simulink model "stm32f0_clcd_demo"  (Simulink 7.3)
settings: Solver=ode3  SolverMode=SingleTasking  StartTime=0.0  StopTime=10.0  RelTol=1e-3
PreLoadFcn:
  | waijung.modelPreload; % Required for working with Waijung Blockset. Do not remove.
undefined symbols (not defined in the file): LQFP48, STM32F072CB
libraries: simulink x34, waijung_soft_i2c_lib x12, waijung_string_manipulate x4, stm32f0_device_config_lib x1
CloseFcn:
  | waijung.modelClose; % Required for working with Waijung Blockset. Do not remove.
settings Model: Creator=Krisada  LastModifiedBy=Krisada
settings OptimizationCC: OptimizeModelRefInitCode=on  LifeSpan=1
settings HardwareCC: ProdEndianess=LittleEndian  ProdHWDeviceType=ARM Compatible->Cortex - M0  TargetEndianess=LittleEndian  TargetHWDeviceType=ARM Compatible->Cortex - M0
settings RTWCC: SystemTargetFile=stm32f0.tlc  GenerateMakefile=off  TemplateMakefile=ert_default_tmf  Description=STM32F0 Target  ProcessScript=stm32f0_make_rtw_hook
settings CodeAppCC: IgnoreCustomStorageClasses=off
settings STFCustomTargetCC: ModelReferenceCompliant=off  CombineOutputUpdateFcns=on  ERTCustomFileBanners=on  SupportContinuousTime=off  SupportNonInlinedSFcns=off  SystemTargetFile=stm32f0.tlc
settings ERTTargetCC: MultiwordLength=2048  ModelReferenceCompliant=off  ParMdlRefBuildCompliant=off  CompOptLevelCompliant=off  ERTFirstTimeCompliant=off  ModelStepFunctionPrototypeControlCompliant=off  CPPClassGenCompliant=off  InlinedParameterPlacement=NonHierarchical  ERTSrcFileBannerTemplate=stm32f0_code_template.cgt  ERTHdrFileBannerTemplate=stm32f0_code_template.cgt  ERTDataSrcFileTemplate=stm32f0_code_template.cgt  ERTDataHdrFileTemplate=stm32f0_code_template.cgt  ERTCustomFileTemplate=stm32f0_file_process.tlc

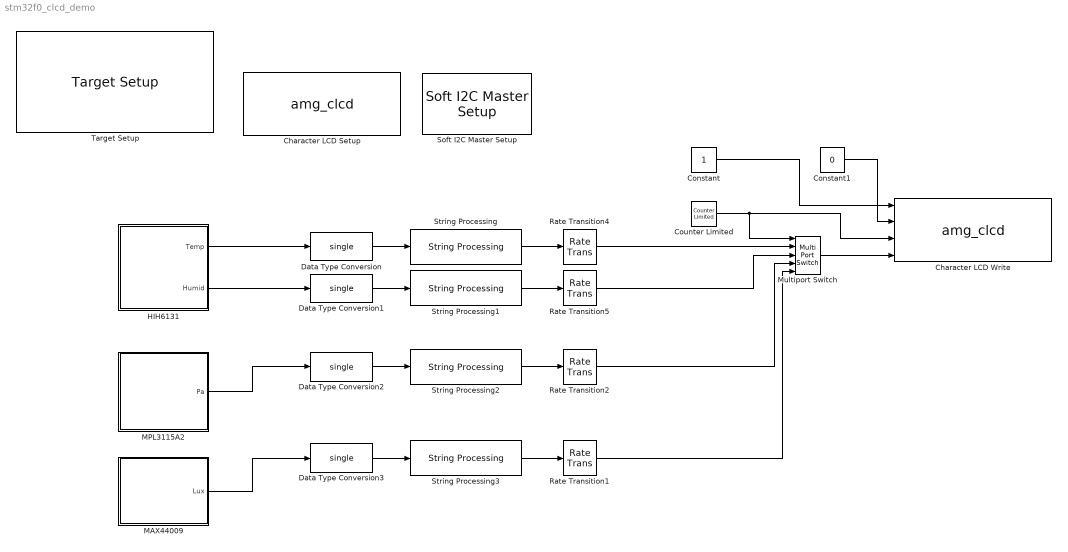
== system stm32f0_clcd_demo ==
  Character LCD Setup : S-Function  FunctionName=amg_clcd  Parameters=module,configuration,inputtypearray,outputtypearray,confstr,sampletime,sampletimestr,blockid  EnableBusSupport=off  mask(amg_clcd){configuration=Setup, module=1, model=amg CLCD Std, interface=4-bits, linecount=4, columncount=16, gpiotype=Push-pull, controlport=B, control_rs=2, control_rw=10, control_en=11, dataport=B, data0=12, data1=13, data2=0, data3=1, usestringbuffer=off, stringbuffer=<empty>, varname=, inputtypearray=[0], outputtypearray=[0], confstr=["4","4","16","PP","B","2","11","10","","B","","","","","12","13","0","1","0","","0","1","0","0","0","0","0","0","0","stm32f0"], sampletime=-1, sampletimestr=0.1, blockid=CharacterLCDSetup}
      mask prompts: model "LCD model:"; linecount "Number of lines (2 or 4):"; columncount "Number of columns (16 or 20):"; gpiotype "GPIO Output type:"; controlport "GPIO control port:"; control_rs "GPIO control pin, RS:"; control_rw "GPIO control pin, RW:"; control_en "GPIO control pin, EN:"; dataport "GPIO data D[7:4] port"; data0 "GPIO data pin, D4:"; data1 "GPIO data pin, D5:"; data2 "GPIO data pin, D6:"; data3 "GPIO data pin, D7:"; usestringbuffer "Use string buffer"; stringbuffer "String buffer"; varname "Variable name"; inputtypearray "Input type array"; outputtypearray "Output type array"; confstr "Configuration string"; sampletime "Sample time (sec)"; sampletimestr "Compiled sample time (sec) in string"
      mask init:
      | amg_clcd_callback('init');
      mask Help: web(fullfile(waijungdocroot,'amg_clcd_setup.htm'), '-browser')
      mask StyleString: popup(Setup|Transaction),popup(1|2|3|4),popup(amg CLCD Std),popup(4-bits),edit,edit,popup(Push-pull|Open-drain),popup(A|B|C|D|E|F|G|H|I),popup(0|1|2|3|4|5|6|7|8|9|10|11|12|13|14|15),popup(0|1|2|3|4|5|6|7|8|9|10|11|12|13|14|15),popup(0|1|2|3|4|5|6|7|8|9|10|11|12|13|14|15),popup(A|B|C|D|E|F|G|H|I),popup(0|1|2|3|4|5|6|7|8|9|10|11|12|13|14|15),popup(0|1|2|3|4|5|6|7|8|9|10|11|12|13|14|15),popup(0|1|2|3|4|5|6|7|8|9|10|11|12|13|14|15),popup(0|1|2|3|4|5|6|7|8|9|10|11|12|13|14|15),checkbox,popup(<empty>),edit,edit,edit,edit,edit,edit,edit
      mask CallbackString: amg_clcd_callback('configuration');||||||||||||||||amg_clcd_callback('usestringbuffer');||amg_clcd_callback('varname');|||amg_clcd_callback('confstr');|amg_clcd_callback('sampletime');|amg_clcd_callback('sampletimestr');|amg_clcd_callback('blockid');
      mask Display: text(0.5, 0.5, 'Module: CLCD1 (Setup)\nInterface: 4-bits\nCntrl: B2/B10/B11\nD[7:4]: B12/B13/B0/B1\nTs (sec): 0.1','ver','middle','hor','center');
  Character LCD Write : S-Function  FunctionName=amg_clcd  Parameters=module,configuration,inputtypearray,outputtypearray,confstr,sampletime,sampletimestr,blockid  EnableBusSupport=off  mask(amg_clcd){configuration=Transaction, module=1, model=amg CLCD Std, interface=4-bits, linecount=4, columncount=20, gpiotype=Push-pull, controlport=E, control_rs=15, control_rw=13, control_en=11, dataport=A, data0=7, data1=5, data2=3, data3=1, usestringbuffer=off, stringbuffer=<empty>, varname=, inputtypearray=[4 -1 -1 -1 -1], outputtypearray=[0], confstr=["4","4","20","PP","E","15","11","13","","A","","","","","7","5","3","1","0","","1","0","0","0","1","0","0","0","0","stm32f0"], sampletime=-1, sampletimestr=0.1, blockid=CharacterLCDWrite}
      mask prompts: model "LCD model:"; linecount "Number of lines:"; columncount "Number of columns:"; gpiotype "GPIO Output type:"; controlport "GPIO control port:"; control_rs "GPIO control pin, RS:"; control_rw "GPIO control pin, RW:"; control_en "GPIO control pin, EN:"; dataport "GPIO data D[7:4] port"; data0 "GPIO data pin, D4:"; data1 "GPIO data pin, D5:"; data2 "GPIO data pin, D6:"; data3 "GPIO data pin, D7:"; usestringbuffer "Use string buffer"; stringbuffer "String buffer"; varname "Variable name"; inputtypearray "Input type array"; outputtypearray "Output type array"; confstr "Configuration string"; sampletime "Sample time (sec)"; sampletimestr "Compiled sample time (sec) in string"
      mask help:
      | Note for cmd:
      | 1 - Clear specified LCD line display before write data to LCD.
      | Otherwise (e.g. 0) - Write data without clearing LCD Line.
      |
      | Position:
      | x = 0, First Character (from left to right)
      | y = 0, Top Line
      mask init:
      | amg_clcd_callback('init');
      mask Help: web(fullfile(waijungdocroot,'amg_clcd_write.htm'), '-browser')
      mask StyleString: popup(Setup|Transaction),popup(1|2|3|4),popup(amg CLCD Std),popup(4-bits),edit,edit,popup(Push-pull|Open-drain),popup(A|B|C|D|E|F|G|H|I),popup(0|1|2|3|4|5|6|7|8|9|10|11|12|13|14|15),popup(0|1|2|3|4|5|6|7|8|9|10|11|12|13|14|15),popup(0|1|2|3|4|5|6|7|8|9|10|11|12|13|14|15),popup(A|B|C|D|E|F|G|H|I),popup(0|1|2|3|4|5|6|7|8|9|10|11|12|13|14|15),popup(0|1|2|3|4|5|6|7|8|9|10|11|12|13|14|15),popup(0|1|2|3|4|5|6|7|8|9|10|11|12|13|14|15),popup(0|1|2|3|4|5|6|7|8|9|10|11|12|13|14|15),checkbox,popup(<empty>),edit,edit,edit,edit,edit,edit,edit
      mask CallbackString: amg_clcd_callback('configuration');||||||||||||||||amg_clcd_callback('usestringbuffer');||amg_clcd_callback('varname');|||amg_clcd_callback('confstr');|amg_clcd_callback('sampletime');|amg_clcd_callback('sampletimestr');|amg_clcd_callback('blockid');
      mask Display: text(0.5, 0.5, 'Module: CLCD1 (Write)\nTs (sec): 0.1','ver','middle','hor','center');port_label('input', 1,'cmd');port_label('input', 2,'xpos');port_label('input', 3,'ypos');port_label('input', 4,'str');
  Constant : Constant  OutDataType=fixdt(1, 16)  OutScaling=2^0
  Constant1 : Constant  Value=0  OutDataType=fixdt(1, 16)  OutScaling=2^0
  Counter Limited : simulink/Sources/Counter Limited  SystemSampleTime=-1  uplimit=3  tsamp=-1
  Data Type Conversion{,1..3} (4 alike) : DataTypeConversion  OutDataTypeMode=single  OutDataType=fixdt(1, 16)  OutScaling=2^0  OutDataTypeStr=single
  HIH6131 : Subsystem
  MAX44009 : Subsystem
  MPL3115A2 : Subsystem
  Multiport Switch : MultiPortSwitch  Inputs=4  zeroidx=on  OutDataType=fixdt(1, 16)  OutScaling=2^0
  Rate Transition{1..2,4..5} (4 alike) : RateTransition
  Soft I2C Master Setup : waijung_soft_i2c_lib/Soft I2C Master Setup  conf=Setup  targetname=stm32f0  module=1  transfer=Blocking  clk=250  timeout=25  sdapins='B7'  sclpins='B6'  writecount=1  readcount=1  waittime=0  forcestop=off  portpinstr=0  sampletime=-1  blockid=SoftI2CMasterSetup  inputporttype=[]  inputportwidth=[]  inputportlabel={}  outputporttype=[]  outputportwidth=[]  outputportlabel={}  compat=0  optionstring="[\"1\",\"250000\",\"3\",\"2\",\"1\",\"1\",\"25\",\"\",\"\",\"\",\"0\",\"1\",\"0\",\"0\",\"0\",\"0\",\"0\",\"0\",\"0\",\"\",\"1\",\"B\",\"7\",\"B\",\"6\"]"
  String Processing : waijung_string_manipulate/String Processing  conf=processing  stringfunction=sprintf  stringformat='Temp:%1.2f'  begindelimiter=''  enddelimiter=''  buffersize=16  enablestatus=off  portpinstr=0  sampletime=inf  blockid=StringProcessing  inputporttype=[-1]  inputportwidth=[1]  inputportlabel={'%f'}  outputporttype=[3]  outputportwidth=[16]  outputportlabel={'Output'}  compat=0  optionstring=[]  datatypestring="[\"float\"]"
  String Processing1 : waijung_string_manipulate/String Processing  conf=processing  stringfunction=sprintf  stringformat='Humid:%1.2f'  begindelimiter=''  enddelimiter=''  buffersize=16  enablestatus=off  portpinstr=0  sampletime=inf  blockid=StringProcessing1  inputporttype=[-1]  inputportwidth=[1]  inputportlabel={'%f'}  outputporttype=[3]  outputportwidth=[16]  outputportlabel={'Output'}  compat=0  optionstring=[]  datatypestring="[\"float\"]"
  String Processing2 : waijung_string_manipulate/String Processing  conf=processing  stringfunction=sprintf  stringformat='Pa: %1.2f'  begindelimiter=''  enddelimiter=''  buffersize=16  enablestatus=off  portpinstr=0  sampletime=inf  blockid=StringProcessing2  inputporttype=[-1]  inputportwidth=[1]  inputportlabel={'%f'}  outputporttype=[3]  outputportwidth=[16]  outputportlabel={'Output'}  compat=0  optionstring=[]  datatypestring="[\"float\"]"
  String Processing3 : waijung_string_manipulate/String Processing  conf=processing  stringfunction=sprintf  stringformat='Lux: %1.2f'  begindelimiter=''  enddelimiter=''  buffersize=16  enablestatus=off  portpinstr=0  sampletime=inf  blockid=StringProcessing3  inputporttype=[-1]  inputportwidth=[1]  inputportlabel={'%f'}  outputporttype=[3]  outputportwidth=[16]  outputportlabel={'Output'}  compat=0  optionstring=[]  datatypestring="[\"float\"]"
  Target Setup : stm32f0_device_config_lib/Target Setup  Priority=100  compiler=GNU ARM  previous_compiler=GNU ARM  mcu=STM32F072CB (LQFP48)  mcustr=STM32F072CB  stdlib=STM32F072  clockconfig=FiO MOTE-ST Default (HSEOSC-8MHz/HCLK-48MHz)  system_stm32f0xx_c_path=F:\trunk\targets\stm32f0_target\stm32f0\utils\STM32F0xx_AN4055\stm32f0_default\hse8mhz_pll_hclk48mhz  showmemoryconfiguration=on  stacksize=0x400  heapsize=0x200  enableautocompiledownload=on  fullchiperase=off  programmerinterface=aMG USB Connect  editctrlstr=on  compilercontrolstr=$(patsubst %, -I%, .) -mcpu=cortex-m0 -mthumb -mabi=aapcs -Wall -O3 -mfloat-abi=soft -ffunction-sections -fdata-sections -fno-strict-aliasing -fno-builtin --short-enums  assemblercontrolstr=$(patsubst %, -I%, .) -mcpu=cortex-m0 -mtune=cortex-m0 -mthumb -Wall -O3 -Wa,-amhls=$(<:.s=.lst) -D__STACK_SIZE=$(STACK_SIZE) -D__HEAP_SIZE=$(HEAP_SIZE)  linkercontrolstr="-T$(LD_SCRIPT) -Wl,-Map=$(MAP),--cref,--no-warn-mismatch -mcpu=cortex-m0 -mthumb  -Wall -O3 -mabi=aapcs -lc -specs=nosys.specs"  runafterdownload=on  execprofile=None  profileruart=3  profilerbaud=500000  profilertxpin=Not used  profilerinitstr=0.1,48000000,4800000,500000,0  manualsetsampletime=off  sampletime=0.1  blockid=TargetSetup  systickreloadvalue=4800000  hseval=8000000  lastprofileruart=3  hclk=48000000  flashorigin=0x8000000  flashlength=128k  ramorigin=0x20000000  ramlength=16k  useextram=off
  wires:
  Data Type Conversion/1 -> String Processing/1
  Data Type Conversion1/1 -> String Processing1/1
  Data Type Conversion3/1 -> String Processing3/1
  String Processing/1 -> Rate Transition4/1
  String Processing1/1 -> Rate Transition5/1
  String Processing3/1 -> Rate Transition1/1
  Counter Limited/1 -> Multiport Switch/1, Character LCD Write/3
  Multiport Switch/1 -> Character LCD Write/4
  Constant/1 -> Character LCD Write/1
  Constant1/1 -> Character LCD Write/2
  Rate Transition4/1 -> Multiport Switch/2
  Rate Transition5/1 -> Multiport Switch/3
  Data Type Conversion2/1 -> String Processing2/1
  String Processing2/1 -> Rate Transition2/1
  Rate Transition2/1 -> Multiport Switch/4
  Rate Transition1/1 -> Multiport Switch/5
  HIH6131/1(Temp) -> Data Type Conversion/1
  HIH6131/2(Humid) -> Data Type Conversion1/1
  MPL3115A2/1(Pa) -> Data Type Conversion2/1
  MAX44009/1(Lux) -> Data Type Conversion3/1

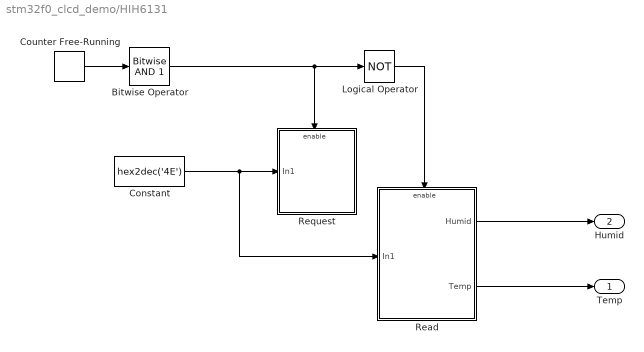
== system stm32f0_clcd_demo/HIH6131 ==
  Bitwise Operator : simulink/Logic and Bit Operations/Bitwise Operator  logicop=AND  UseBitMask=on  BitMask=1  BitMaskRealWorld=Stored Integer
  Constant : Constant  Value=hex2dec('4E')  OutDataTypeMode=uint8  OutDataType=fixdt(1, 16)  OutScaling=2^0  OutDataTypeStr=uint8  SampleTime=0.5
  Counter Free-Running : simulink/Sources/Counter Free-Running  SystemSampleTime=-1  NumBits=16  tsamp=-1
  Logical Operator : Logic  Operator=NOT  AllPortsSameDT=off  OutDataTypeMode=boolean  LogicDataType=fixdt(0, 8)  OutDataTypeStr=boolean
  Read : Subsystem
  Request : Subsystem
  Temp : Outport
  Humid : Outport  Port=2
  wires:
  Constant/1 -> Read/1(In1), Request/1(In1)
  Counter Free-Running/1 -> Bitwise Operator/1
  Bitwise Operator/1 -> Logical Operator/1, Request/Enable
  Logical Operator/1 -> Read/Enable
  Read/1(Humid) -> Humid/1
  Read/2(Temp) -> Temp/1

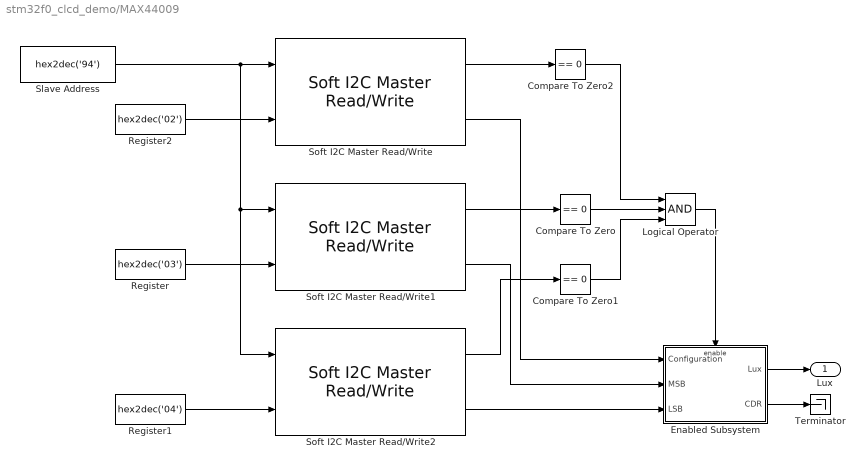
== system stm32f0_clcd_demo/MAX44009 ==
  Compare To Zero : simulink/Logic and Bit Operations/Compare To Zero  SystemSampleTime=-1  relop===  LogicOutDataTypeMode=uint8  ZeroCross=off
  Compare To Zero1 : simulink/Logic and Bit Operations/Compare To Zero  SystemSampleTime=-1  relop===  LogicOutDataTypeMode=uint8  ZeroCross=off
  Compare To Zero2 : simulink/Logic and Bit Operations/Compare To Zero  SystemSampleTime=-1  relop===  LogicOutDataTypeMode=uint8  ZeroCross=off
  Enabled Subsystem : Subsystem  TreatAsAtomicUnit=on
  Logical Operator : Logic  Inputs=3  AllPortsSameDT=off  OutDataTypeMode=boolean  LogicDataType=fixdt(0, 8)  OutDataTypeStr=boolean
  Register : Constant  Value=hex2dec('03')  OutDataTypeMode=uint8  OutDataType=fixdt(1, 16)  OutScaling=2^0  OutDataTypeStr=uint8
  Register1 : Constant  Value=hex2dec('04')  OutDataTypeMode=uint8  OutDataType=fixdt(1, 16)  OutScaling=2^0  OutDataTypeStr=uint8
  Register2 : Constant  Value=hex2dec('02')  OutDataTypeMode=uint8  OutDataType=fixdt(1, 16)  OutScaling=2^0  OutDataTypeStr=uint8
  Slave Address : Constant  Value=hex2dec('94')  OutDataTypeMode=uint8  OutDataType=fixdt(1, 16)  OutScaling=2^0  OutDataTypeStr=uint8  SampleTime=0.5
  Soft I2C Master Read/Write : waijung_soft_i2c_lib/Soft I2C Master Read//Write  conf=ReadWrite  targetname=stm32f0  module=1  transfer=Blocking  clk=100  timeout=25  sdapins={'A4','A6'}  sclpins='A5'  writecount=1  readcount=1  waittime=0  forcestop=off  portpinstr=0  sampletime=inf  blockid=MAX44009SoftI2CMasterReadWrite  inputporttype=[3 3]  inputportwidth=[]  inputportlabel={'SlvAddr' 'Wr0 (uint8)'}  outputporttype=[3 3 ]  outputportwidth=[1 1]  outputportlabel={'Status' 'Rd0 (uint8)'}  compat=0  optionstring="[\"1\",\"1\",\"1\",\"0\",\"off\",\"1\"]"
  Soft I2C Master Read/Write1 : waijung_soft_i2c_lib/Soft I2C Master Read//Write  conf=ReadWrite  targetname=stm32f0  module=1  transfer=Blocking  clk=100  timeout=25  sdapins={'A4','A6'}  sclpins='A5'  writecount=1  readcount=1  waittime=0  forcestop=off  portpinstr=0  sampletime=inf  blockid=MAX44009SoftI2CMasterReadWrite1  inputporttype=[3 3]  inputportwidth=[]  inputportlabel={'SlvAddr' 'Wr0 (uint8)'}  outputporttype=[3 3 ]  outputportwidth=[1 1]  outputportlabel={'Status' 'Rd0 (uint8)'}  compat=0  optionstring="[\"1\",\"1\",\"1\",\"0\",\"off\",\"1\"]"
  Soft I2C Master Read/Write2 : waijung_soft_i2c_lib/Soft I2C Master Read//Write  conf=ReadWrite  targetname=stm32f0  module=1  transfer=Blocking  clk=100  timeout=25  sdapins={'A4','A6'}  sclpins='A5'  writecount=1  readcount=1  waittime=0  forcestop=off  portpinstr=0  sampletime=inf  blockid=MAX44009SoftI2CMasterReadWrite2  inputporttype=[3 3]  inputportwidth=[]  inputportlabel={'SlvAddr' 'Wr0 (uint8)'}  outputporttype=[3 3 ]  outputportwidth=[1 1]  outputportlabel={'Status' 'Rd0 (uint8)'}  compat=0  optionstring="[\"1\",\"1\",\"1\",\"0\",\"off\",\"1\"]"
  Terminator : Terminator
  Lux : Outport  OutDataType=fixdt(1, 16)  OutScaling=2^0
  wires:
  Enabled Subsystem/2(CDR) -> Terminator/1
  Enabled Subsystem/1(Lux) -> Lux/1
  Soft I2C Master Read/Write1/1 -> Compare To Zero/1
  Register/1 -> Soft I2C Master Read/Write1/2
  Slave Address/1 -> Soft I2C Master Read/Write1/1, Soft I2C Master Read/Write2/1, Soft I2C Master Read/Write/1
  Register1/1 -> Soft I2C Master Read/Write2/2
  Soft I2C Master Read/Write2/1 -> Compare To Zero1/1
  Logical Operator/1 -> Enabled Subsystem/Enable
  Soft I2C Master Read/Write1/2 -> Enabled Subsystem/2(MSB)
  Soft I2C Master Read/Write2/2 -> Enabled Subsystem/3(LSB)
  Register2/1 -> Soft I2C Master Read/Write/2
  Soft I2C Master Read/Write/1 -> Compare To Zero2/1
  Compare To Zero/1 -> Logical Operator/2
  Compare To Zero2/1 -> Logical Operator/1
  Compare To Zero1/1 -> Logical Operator/3
  Soft I2C Master Read/Write/2 -> Enabled Subsystem/1(Configuration)

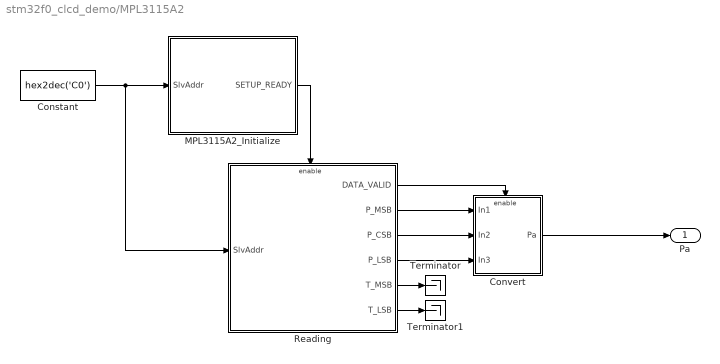
== system stm32f0_clcd_demo/MPL3115A2 ==
  Constant : Constant  Value=hex2dec('C0')  OutDataTypeMode=uint8  OutDataType=fixdt(1, 16)  OutScaling=2^0  OutDataTypeStr=uint8  SampleTime=0.5
  Convert : Subsystem
  MPL3115A2_Initialize : Subsystem
  Reading : Subsystem  TreatAsAtomicUnit=on
  Terminator : Terminator
  Terminator1 : Terminator
  Pa : Outport
  wires:
  Constant/1 -> MPL3115A2_Initialize/1(SlvAddr), Reading/1(SlvAddr)
  Reading/1(DATA_VALID) -> Convert/Enable
  Reading/6(T_LSB) -> Terminator1/1
  Reading/5(T_MSB) -> Terminator/1
  Reading/4(P_LSB) -> Convert/3(In3)
  Reading/3(P_CSB) -> Convert/2(In2)
  Reading/2(P_MSB) -> Convert/1(In1)
  MPL3115A2_Initialize/1(SETUP_READY) -> Reading/Enable
  Convert/1(Pa) -> Pa/1

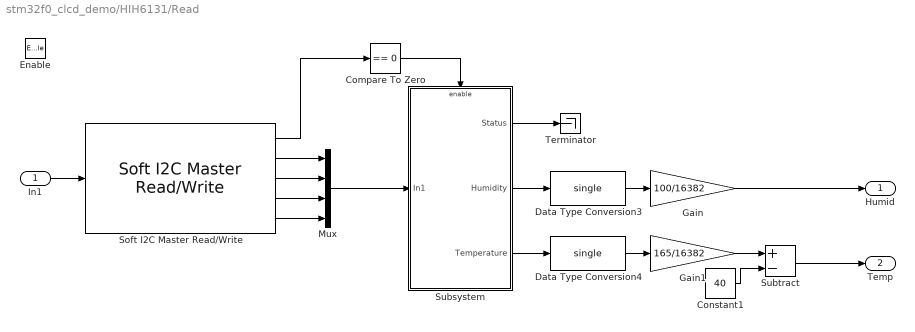
== system stm32f0_clcd_demo/HIH6131/Read ==
  In1 : Inport
  Enable : EnablePort
  Compare To Zero : simulink/Logic and Bit Operations/Compare To Zero  SystemSampleTime=-1  relop===  LogicOutDataTypeMode=boolean  ZeroCross=off
  Constant1 : Constant  Value=40  OutDataTypeMode=single  OutDataType=fixdt(1, 16)  OutScaling=2^0  OutDataTypeStr=single
  Data Type Conversion3 : DataTypeConversion  OutDataTypeMode=single  OutDataType=fixdt(1, 16)  OutScaling=2^0  OutDataTypeStr=single
  Data Type Conversion4 : DataTypeConversion  OutDataTypeMode=single  OutDataType=fixdt(1, 16)  OutScaling=2^0  OutDataTypeStr=single
  Gain : Gain  Gain=100/16382  ParameterDataType=fixdt(1, 16)  ParameterScaling=2^0  OutDataType=fixdt(1, 16)  OutScaling=2^0
  Gain1 : Gain  Gain=165/16382  ParameterDataType=fixdt(1, 16)  ParameterScaling=2^0  OutDataType=fixdt(1, 16)  OutScaling=2^0
  Mux : Mux
  Soft I2C Master Read/Write : waijung_soft_i2c_lib/Soft I2C Master Read//Write  conf=ReadWrite  targetname=stm32f0  module=1  transfer=Blocking  clk=100  timeout=25  sdapins={'A4','A6'}  sclpins='A5'  writecount=0  readcount=4  waittime=0  forcestop=off  portpinstr=0  sampletime=inf  blockid=HIH6131ReadSoftI2CMasterReadWrite  inputporttype=[3]  inputportwidth=[]  inputportlabel={'SlvAddr'}  outputporttype="[3 3 3 3 3    ]"  outputportwidth=[1 1 1 1 1]  outputportlabel={'Status' 'Rd0 (uint8)' 'Rd1 (uint8)' 'Rd2 (uint8)' 'Rd3 (uint8)'}  compat=0  optionstring="[\"1\",\"0\",\"4\",\"0\",\"off\",\"1\"]"
  Subsystem : Subsystem
  Subtract : Sum  Inputs=+-  OutDataType=fixdt(1, 16)  OutScaling=2^-10
  Terminator : Terminator
  Humid : Outport  OutDataType=fixdt(1, 16)  OutScaling=2^0
  Temp : Outport  Port=2  OutDataType=fixdt(1, 16)  OutScaling=2^0
  wires:
  Soft I2C Master Read/Write/2 -> Mux/1
  Soft I2C Master Read/Write/3 -> Mux/2
  Soft I2C Master Read/Write/4 -> Mux/3
  Soft I2C Master Read/Write/5 -> Mux/4
  Mux/1 -> Subsystem/1(In1)
  Compare To Zero/1 -> Subsystem/Enable
  Soft I2C Master Read/Write/1 -> Compare To Zero/1
  Subsystem/2(Humidity) -> Data Type Conversion3/1
  Subsystem/3(Temperature) -> Data Type Conversion4/1
  Gain1/1 -> Subtract/1
  Constant1/1 -> Subtract/2
  Subsystem/1(Status) -> Terminator/1
  Subtract/1 -> Temp/1
  Data Type Conversion3/1 -> Gain/1
  Data Type Conversion4/1 -> Gain1/1
  Gain/1 -> Humid/1
  In1/1 -> Soft I2C Master Read/Write/1

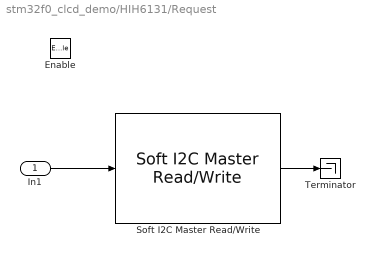
== system stm32f0_clcd_demo/HIH6131/Request ==
  In1 : Inport
  Enable : EnablePort
  Soft I2C Master Read/Write : waijung_soft_i2c_lib/Soft I2C Master Read//Write  conf=ReadWrite  targetname=stm32f0  module=1  transfer=Blocking  clk=100  timeout=25  sdapins={'A4','A6'}  sclpins='A5'  writecount=0  readcount=0  waittime=0  forcestop=off  portpinstr=0  sampletime=inf  blockid=HIH6131RequestSoftI2CMasterReadWrite  inputporttype=[3]  inputportwidth=[]  inputportlabel={'SlvAddr'}  outputporttype=[3]  outputportwidth=[1]  outputportlabel={'Status'}  compat=0  optionstring="[\"1\",\"0\",\"0\",\"0\",\"off\",\"1\"]"
  Terminator : Terminator
  wires:
  In1/1 -> Soft I2C Master Read/Write/1
  Soft I2C Master Read/Write/1 -> Terminator/1

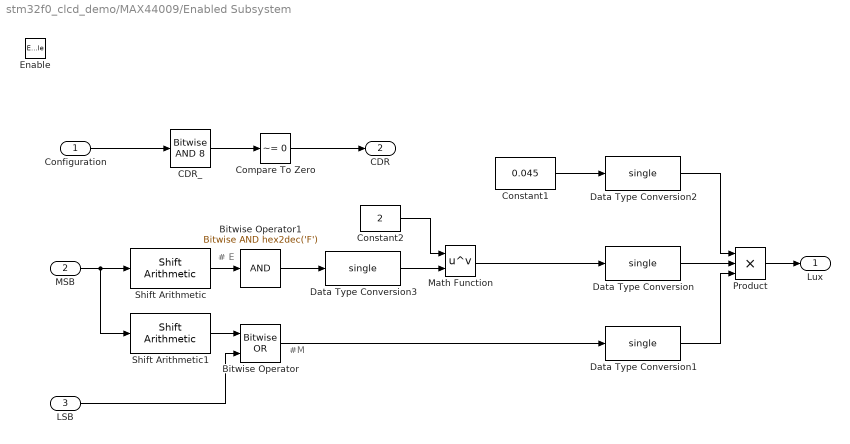
== system stm32f0_clcd_demo/MAX44009/Enabled Subsystem ==
  note: # E
  note: #M
  Configuration : Inport  OutDataType=fixdt(1, 16)  OutScaling=2^0
  MSB : Inport  Port=2  OutDataType=fixdt(1, 16)  OutScaling=2^0
  LSB : Inport  Port=3  OutDataType=fixdt(1, 16)  OutScaling=2^0
  Enable : EnablePort
  Bitwise Operator : simulink/Logic and Bit Operations/Bitwise Operator  logicop=OR  UseBitMask=off  NumInputPorts=2  BitMask=bin2dec('11011001')  BitMaskRealWorld=Stored Integer
  Bitwise Operator1 : simulink/Logic and Bit Operations/Bitwise Operator  logicop=AND  UseBitMask=on  BitMask=hex2dec('F')  BitMaskRealWorld=Stored Integer
  CDR_ : simulink/Logic and Bit Operations/Bitwise Operator  logicop=AND  UseBitMask=on  BitMask=8  BitMaskRealWorld=Stored Integer
  Compare To Zero : simulink/Logic and Bit Operations/Compare To Zero  SystemSampleTime=-1  relop=~=  LogicOutDataTypeMode=uint8  ZeroCross=off
  Constant1 : Constant  Value=0.045  OutDataType=fixdt(1, 16)  OutScaling=2^0
  Constant2 : Constant  Value=2  OutDataTypeMode=single  OutDataType=fixdt(1, 16)  OutScaling=2^0  OutDataTypeStr=single
  Data Type Conversion{,1..3} (4 alike) : DataTypeConversion  OutDataTypeMode=single  OutDataType=fixdt(1, 16)  OutScaling=2^0  OutDataTypeStr=single
  Math Function : Math  Operator=pow  OutDataType=fixdt(1, 16)  OutScaling=2^0  SaturateOnIntegerOverflow=on
  Product : Product  Inputs=3  OutDataType=fixdt(1, 16)  OutScaling=2^0  RndMeth=Zero  OutDataTypeStr=Inherit: Same as first input
  Shift Arithmetic : simulink/Logic and Bit Operations/Shift Arithmetic  SystemSampleTime=-1  nBitShiftRight=4  nBinPtShiftRight=0
  Shift Arithmetic1 : simulink/Logic and Bit Operations/Shift Arithmetic  SystemSampleTime=-1  nBitShiftRight=-4  nBinPtShiftRight=0
  Lux : Outport  OutDataType=fixdt(1, 16)  OutScaling=2^0
  CDR : Outport  Port=2  OutDataType=fixdt(1, 16)  OutScaling=2^0
  wires:
  Compare To Zero/1 -> CDR/1
  CDR_/1 -> Compare To Zero/1
  Data Type Conversion2/1 -> Product/1
  Data Type Conversion/1 -> Product/2
  Bitwise Operator1/1 -> Data Type Conversion3/1
  Constant1/1 -> Data Type Conversion2/1
  Math Function/1 -> Data Type Conversion/1
  MSB/1 -> Shift Arithmetic/1, Shift Arithmetic1/1
  Shift Arithmetic/1 -> Bitwise Operator1/1
  Shift Arithmetic1/1 -> Bitwise Operator/1
  LSB/1 -> Bitwise Operator/2
  Bitwise Operator/1 -> Data Type Conversion1/1
  Data Type Conversion1/1 -> Product/3
  Configuration/1 -> CDR_/1
  Product/1 -> Lux/1
  Constant2/1 -> Math Function/1
  Data Type Conversion3/1 -> Math Function/2

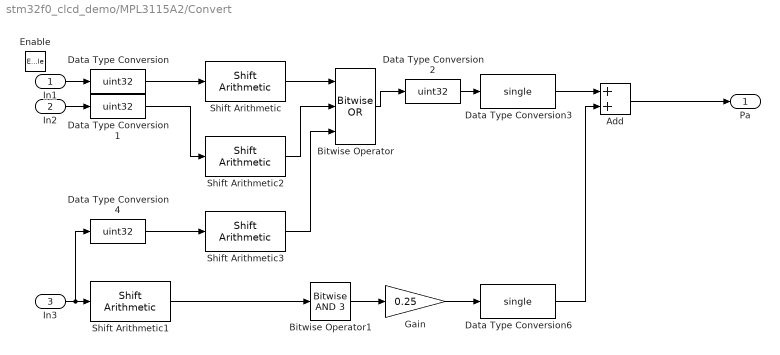
== system stm32f0_clcd_demo/MPL3115A2/Convert ==
  In1 : Inport
  In2 : Inport  Port=2
  In3 : Inport  Port=3
  Enable : EnablePort
  Add : Sum  OutDataType=fixdt(1, 16)  OutScaling=2^-10
  Bitwise Operator : simulink/Logic and Bit Operations/Bitwise Operator  logicop=OR  UseBitMask=off  NumInputPorts=3  BitMask=bin2dec('11011001')  BitMaskRealWorld=Stored Integer
  Bitwise Operator1 : simulink/Logic and Bit Operations/Bitwise Operator  logicop=AND  UseBitMask=on  BitMask=3  BitMaskRealWorld=Stored Integer
  Data Type Conversion{,1..2,4} (4 alike) : DataTypeConversion  OutDataTypeMode=uint32  OutDataType=fixdt(1, 16)  OutScaling=2^0  OutDataTypeStr=uint32
  Data Type Conversion3 : DataTypeConversion  OutDataTypeMode=single  OutDataType=fixdt(1, 16)  OutScaling=2^0  OutDataTypeStr=single
  Data Type Conversion6 : DataTypeConversion  OutDataTypeMode=single  OutDataType=fixdt(1, 16)  OutScaling=2^0  OutDataTypeStr=single
  Gain : Gain  Gain=0.25  ParameterDataType=fixdt(1, 16)  ParameterScaling=2^0  OutDataTypeMode=single  OutDataType=fixdt(1, 16)  OutScaling=2^0  OutDataTypeStr=single
  Shift Arithmetic : simulink/Logic and Bit Operations/Shift Arithmetic  SystemSampleTime=-1  nBitShiftRight=-10  nBinPtShiftRight=0
  Shift Arithmetic1 : simulink/Logic and Bit Operations/Shift Arithmetic  SystemSampleTime=-1  nBitShiftRight=4  nBinPtShiftRight=0
  Shift Arithmetic2 : simulink/Logic and Bit Operations/Shift Arithmetic  SystemSampleTime=-1  nBitShiftRight=-2  nBinPtShiftRight=0
  Shift Arithmetic3 : simulink/Logic and Bit Operations/Shift Arithmetic  SystemSampleTime=-1  nBitShiftRight=6  nBinPtShiftRight=0
  Pa : Outport  OutDataType=fixdt(1, 16)  OutScaling=2^0
  wires:
  Shift Arithmetic3/1 -> Bitwise Operator/3
  Data Type Conversion4/1 -> Shift Arithmetic3/1
  Shift Arithmetic2/1 -> Bitwise Operator/2
  In3/1 -> Data Type Conversion4/1, Shift Arithmetic1/1
  In2/1 -> Data Type Conversion1/1
  Add/1 -> Pa/1
  In1/1 -> Data Type Conversion/1
  Data Type Conversion6/1 -> Add/2
  Gain/1 -> Data Type Conversion6/1
  Data Type Conversion3/1 -> Add/1
  Bitwise Operator1/1 -> Gain/1
  Shift Arithmetic1/1 -> Bitwise Operator1/1
  Data Type Conversion2/1 -> Data Type Conversion3/1
  Bitwise Operator/1 -> Data Type Conversion2/1
  Data Type Conversion1/1 -> Shift Arithmetic2/1
  Shift Arithmetic/1 -> Bitwise Operator/1
  Data Type Conversion/1 -> Shift Arithmetic/1

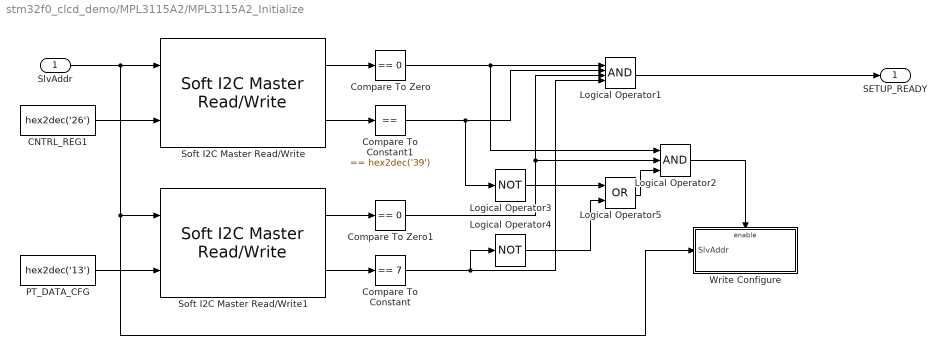
== system stm32f0_clcd_demo/MPL3115A2/MPL3115A2_Initialize ==
  SlvAddr : Inport  OutDataType=fixdt(1, 16)  OutScaling=2^0
  CNTRL_REG1 : Constant  Value=hex2dec('26')  OutDataTypeMode=uint8  OutDataType=fixdt(1, 16)  OutScaling=2^0  OutDataTypeStr=uint8
  Compare To Constant : simulink/Logic and Bit Operations/Compare To Constant  SystemSampleTime=-1  relop===  const=7  LogicOutDataTypeMode=boolean  ZeroCross=off
  Compare To Constant1 : simulink/Logic and Bit Operations/Compare To Constant  SystemSampleTime=-1  relop===  const=hex2dec('39')  LogicOutDataTypeMode=boolean  ZeroCross=off
  Compare To Zero : simulink/Logic and Bit Operations/Compare To Zero  SystemSampleTime=-1  relop===  LogicOutDataTypeMode=boolean  ZeroCross=off
  Compare To Zero1 : simulink/Logic and Bit Operations/Compare To Zero  SystemSampleTime=-1  relop===  LogicOutDataTypeMode=boolean  ZeroCross=off
  Logical Operator1 : Logic  Inputs=4  AllPortsSameDT=off  OutDataTypeMode=boolean  LogicDataType=fixdt(0, 8)  OutDataTypeStr=boolean
  Logical Operator2 : Logic  Inputs=3  AllPortsSameDT=off  OutDataTypeMode=boolean  LogicDataType=fixdt(0, 8)  OutDataTypeStr=boolean
  Logical Operator3 : Logic  Operator=NOT  Inputs=4  AllPortsSameDT=off  OutDataTypeMode=boolean  LogicDataType=fixdt(0, 8)  OutDataTypeStr=boolean
  Logical Operator4 : Logic  Operator=NOT  Inputs=4  AllPortsSameDT=off  OutDataTypeMode=boolean  LogicDataType=fixdt(0, 8)  OutDataTypeStr=boolean
  Logical Operator5 : Logic  Operator=OR  AllPortsSameDT=off  OutDataTypeMode=boolean  LogicDataType=fixdt(0, 8)  OutDataTypeStr=boolean
  PT_DATA_CFG : Constant  Value=hex2dec('13')  OutDataTypeMode=uint8  OutDataType=fixdt(1, 16)  OutScaling=2^0  OutDataTypeStr=uint8
  Soft I2C Master Read/Write : waijung_soft_i2c_lib/Soft I2C Master Read//Write  conf=ReadWrite  targetname=stm32f0  module=1  transfer=Blocking  clk=100  timeout=25  sdapins={'A4','A6'}  sclpins='A5'  writecount=1  readcount=1  waittime=0  forcestop=off  portpinstr=0  sampletime=inf  blockid=MPL3115A2MPL3115A2_InitializeSoftI2CMasterReadWrite  inputporttype=[3 3]  inputportwidth=[]  inputportlabel={'SlvAddr' 'Wr0 (uint8)'}  outputporttype=[3 3 ]  outputportwidth=[1 1]  outputportlabel={'Status' 'Rd0 (uint8)'}  compat=0  optionstring="[\"1\",\"1\",\"1\",\"0\",\"off\",\"1\"]"
  Soft I2C Master Read/Write1 : waijung_soft_i2c_lib/Soft I2C Master Read//Write  conf=ReadWrite  targetname=stm32f0  module=1  transfer=Blocking  clk=100  timeout=25  sdapins={'A4','A6'}  sclpins='A5'  writecount=1  readcount=1  waittime=0  forcestop=off  portpinstr=0  sampletime=inf  blockid=MPL3115A2MPL3115A2_InitializeSoftI2CMasterReadWrite1  inputporttype=[3 3]  inputportwidth=[]  inputportlabel={'SlvAddr' 'Wr0 (uint8)'}  outputporttype=[3 3 ]  outputportwidth=[1 1]  outputportlabel={'Status' 'Rd0 (uint8)'}  compat=0  optionstring="[\"1\",\"1\",\"1\",\"0\",\"off\",\"1\"]"
  Write Configure : Subsystem  TreatAsAtomicUnit=on
  SETUP_READY : Outport  OutDataType=fixdt(1, 16)  OutScaling=2^0
  wires:
  Logical Operator1/1 -> SETUP_READY/1
  Logical Operator5/1 -> Logical Operator2/3
  Logical Operator3/1 -> Logical Operator5/1
  Logical Operator4/1 -> Logical Operator5/2
  Logical Operator2/1 -> Write Configure/Enable
  Compare To Constant/1 -> Logical Operator4/1, Logical Operator1/4
  Compare To Zero1/1 -> Logical Operator2/2, Logical Operator1/3
  Compare To Constant1/1 -> Logical Operator3/1, Logical Operator1/2
  Soft I2C Master Read/Write/2 -> Compare To Constant1/1
  Soft I2C Master Read/Write1/2 -> Compare To Constant/1
  Compare To Zero/1 -> Logical Operator2/1, Logical Operator1/1
  Soft I2C Master Read/Write1/1 -> Compare To Zero1/1
  Soft I2C Master Read/Write/1 -> Compare To Zero/1
  PT_DATA_CFG/1 -> Soft I2C Master Read/Write1/2
  CNTRL_REG1/1 -> Soft I2C Master Read/Write/2
  SlvAddr/1 -> Write Configure/1(SlvAddr), Soft I2C Master Read/Write1/1, Soft I2C Master Read/Write/1

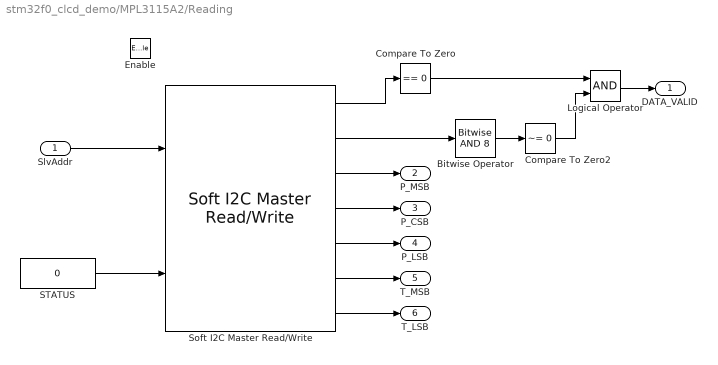
== system stm32f0_clcd_demo/MPL3115A2/Reading ==
  SlvAddr : Inport  OutDataType=fixdt(1, 16)  OutScaling=2^0
  Enable : EnablePort
  Bitwise Operator : simulink/Logic and Bit Operations/Bitwise Operator  logicop=AND  UseBitMask=on  BitMask=8  BitMaskRealWorld=Stored Integer
  Compare To Zero : simulink/Logic and Bit Operations/Compare To Zero  SystemSampleTime=-1  relop===  LogicOutDataTypeMode=boolean  ZeroCross=off
  Compare To Zero2 : simulink/Logic and Bit Operations/Compare To Zero  SystemSampleTime=-1  relop=~=  LogicOutDataTypeMode=boolean  ZeroCross=off
  Logical Operator : Logic  AllPortsSameDT=off  OutDataTypeMode=boolean  LogicDataType=fixdt(0, 8)  OutDataTypeStr=boolean
  STATUS : Constant  Value=0  OutDataTypeMode=uint8  OutDataType=fixdt(1, 16)  OutScaling=2^0  OutDataTypeStr=uint8
  Soft I2C Master Read/Write : waijung_soft_i2c_lib/Soft I2C Master Read//Write  conf=ReadWrite  targetname=stm32f0  module=1  transfer=Blocking  clk=100  timeout=25  sdapins={'A4','A6'}  sclpins='A5'  writecount=1  readcount=6  waittime=0  forcestop=off  portpinstr=0  sampletime=inf  blockid=MPL3115A2ReadingSoftI2CMasterReadWrite  inputporttype=[3 3]  inputportwidth=[]  inputportlabel={'SlvAddr' 'Wr0 (uint8)'}  outputporttype="[3 3 3 3 3 3 3      ]"  outputportwidth=[1 1 1 1 1 1 1]  outputportlabel={'Status' 'Rd0 (uint8)' 'Rd1 (uint8)' 'Rd2 (uint8)' 'Rd3 (uint8)' 'Rd4 (uint8)' 'Rd5 (uint8)'}  compat=0  optionstring="[\"1\",\"1\",\"6\",\"0\",\"off\",\"1\"]"
  DATA_VALID : Outport  OutDataType=fixdt(1, 16)  OutScaling=2^0
  P_MSB : Outport  Port=2  OutDataType=fixdt(1, 16)  OutScaling=2^0
  P_CSB : Outport  Port=3  OutDataType=fixdt(1, 16)  OutScaling=2^0
  P_LSB : Outport  Port=4  OutDataType=fixdt(1, 16)  OutScaling=2^0
  T_MSB : Outport  Port=5  OutDataType=fixdt(1, 16)  OutScaling=2^0
  T_LSB : Outport  Port=6  OutDataType=fixdt(1, 16)  OutScaling=2^0
  wires:
  Soft I2C Master Read/Write/7 -> T_LSB/1
  Soft I2C Master Read/Write/6 -> T_MSB/1
  Soft I2C Master Read/Write/5 -> P_LSB/1
  Soft I2C Master Read/Write/4 -> P_CSB/1
  Soft I2C Master Read/Write/3 -> P_MSB/1
  Compare To Zero/1 -> Logical Operator/1
  Soft I2C Master Read/Write/2 -> Bitwise Operator/1
  Soft I2C Master Read/Write/1 -> Compare To Zero/1
  Logical Operator/1 -> DATA_VALID/1
  Compare To Zero2/1 -> Logical Operator/2
  Bitwise Operator/1 -> Compare To Zero2/1
  STATUS/1 -> Soft I2C Master Read/Write/2
  SlvAddr/1 -> Soft I2C Master Read/Write/1

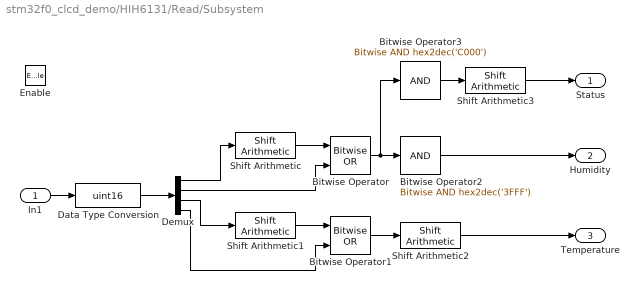
== system stm32f0_clcd_demo/HIH6131/Read/Subsystem ==
  In1 : Inport
  Enable : EnablePort
  Bitwise Operator : simulink/Logic and Bit Operations/Bitwise Operator  logicop=OR  UseBitMask=off  NumInputPorts=2  BitMask=bin2dec('11011001')  BitMaskRealWorld=Stored Integer
  Bitwise Operator1 : simulink/Logic and Bit Operations/Bitwise Operator  logicop=OR  UseBitMask=off  NumInputPorts=2  BitMask=bin2dec('11011001')  BitMaskRealWorld=Stored Integer
  Bitwise Operator2 : simulink/Logic and Bit Operations/Bitwise Operator  logicop=AND  UseBitMask=on  BitMask=hex2dec('3FFF')  BitMaskRealWorld=Stored Integer
  Bitwise Operator3 : simulink/Logic and Bit Operations/Bitwise Operator  logicop=AND  UseBitMask=on  BitMask=hex2dec('C000')  BitMaskRealWorld=Stored Integer
  Data Type Conversion : DataTypeConversion  OutDataTypeMode=uint16  OutDataType=fixdt(1, 16)  OutScaling=2^0  OutDataTypeStr=uint16
  Demux : Demux
  Shift Arithmetic : simulink/Logic and Bit Operations/Shift Arithmetic  SystemSampleTime=-1  nBitShiftRight=-8  nBinPtShiftRight=0
  Shift Arithmetic1 : simulink/Logic and Bit Operations/Shift Arithmetic  SystemSampleTime=-1  nBitShiftRight=-8  nBinPtShiftRight=0
  Shift Arithmetic2 : simulink/Logic and Bit Operations/Shift Arithmetic  SystemSampleTime=-1  nBitShiftRight=2  nBinPtShiftRight=0
  Shift Arithmetic3 : simulink/Logic and Bit Operations/Shift Arithmetic  SystemSampleTime=-1  nBitShiftRight=14  nBinPtShiftRight=0
  Status : Outport
  Humidity : Outport  Port=2
  Temperature : Outport  Port=3
  wires:
  Data Type Conversion/1 -> Demux/1
  Demux/1 -> Shift Arithmetic/1
  Shift Arithmetic/1 -> Bitwise Operator/1
  Demux/2 -> Bitwise Operator/2
  Demux/3 -> Shift Arithmetic1/1
  Shift Arithmetic1/1 -> Bitwise Operator1/1
  Demux/4 -> Bitwise Operator1/2
  Bitwise Operator/1 -> Bitwise Operator2/1, Bitwise Operator3/1
  Bitwise Operator1/1 -> Shift Arithmetic2/1
  Bitwise Operator3/1 -> Shift Arithmetic3/1
  Shift Arithmetic3/1 -> Status/1
  Bitwise Operator2/1 -> Humidity/1
  In1/1 -> Data Type Conversion/1
  Shift Arithmetic2/1 -> Temperature/1

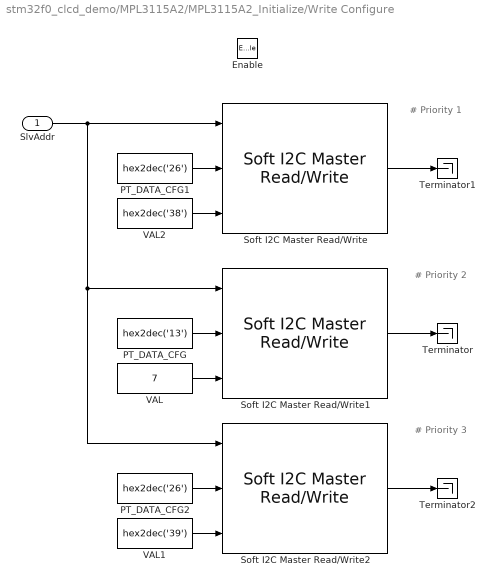
== system stm32f0_clcd_demo/MPL3115A2/MPL3115A2_Initialize/Write Configure ==
  note: # Priority 3
  note: # Priority 2
  note: # Priority 1
  SlvAddr : Inport  OutDataType=fixdt(1, 16)  OutScaling=2^0
  Enable : EnablePort
  PT_DATA_CFG : Constant  Value=hex2dec('13')  OutDataTypeMode=uint8  OutDataType=fixdt(1, 16)  OutScaling=2^0  OutDataTypeStr=uint8
  PT_DATA_CFG1 : Constant  Value=hex2dec('26')  OutDataTypeMode=uint8  OutDataType=fixdt(1, 16)  OutScaling=2^0  OutDataTypeStr=uint8
  PT_DATA_CFG2 : Constant  Value=hex2dec('26')  OutDataTypeMode=uint8  OutDataType=fixdt(1, 16)  OutScaling=2^0  OutDataTypeStr=uint8
  Soft I2C Master Read/Write : waijung_soft_i2c_lib/Soft I2C Master Read//Write  conf=ReadWrite  targetname=stm32f0  module=1  transfer=Blocking  clk=100  timeout=25  sdapins={'A4','A6'}  sclpins='A5'  writecount=2  readcount=0  waittime=0  forcestop=off  portpinstr=0  sampletime=inf  blockid=MPL3115A2MPL3115A2_InitializeWriteConfigureSoftI2CMasterReadWrite  inputporttype=[3 3 3]  inputportwidth=[]  inputportlabel={'SlvAddr' 'Wr0 (uint8)' 'Wr1 (uint8)'}  outputporttype=[3]  outputportwidth=[1]  outputportlabel={'Status'}  compat=0  optionstring="[\"1\",\"2\",\"0\",\"0\",\"off\",\"1\"]"
  Soft I2C Master Read/Write1 : waijung_soft_i2c_lib/Soft I2C Master Read//Write  conf=ReadWrite  targetname=stm32f0  module=1  transfer=Blocking  clk=100  timeout=25  sdapins={'A4','A6'}  sclpins='A5'  writecount=2  readcount=0  waittime=0  forcestop=off  portpinstr=0  sampletime=inf  blockid=MPL3115A2MPL3115A2_InitializeWriteConfigureSoftI2CMasterReadWrite1  inputporttype=[3 3 3]  inputportwidth=[]  inputportlabel={'SlvAddr' 'Wr0 (uint8)' 'Wr1 (uint8)'}  outputporttype=[3]  outputportwidth=[1]  outputportlabel={'Status'}  compat=0  optionstring="[\"1\",\"2\",\"0\",\"0\",\"off\",\"1\"]"
  Soft I2C Master Read/Write2 : waijung_soft_i2c_lib/Soft I2C Master Read//Write  conf=ReadWrite  targetname=stm32f0  module=1  transfer=Blocking  clk=100  timeout=25  sdapins={'A4','A6'}  sclpins='A5'  writecount=2  readcount=0  waittime=0  forcestop=off  portpinstr=0  sampletime=inf  blockid=MPL3115A2MPL3115A2_InitializeWriteConfigureSoftI2CMasterReadWrite2  inputporttype=[3 3 3]  inputportwidth=[]  inputportlabel={'SlvAddr' 'Wr0 (uint8)' 'Wr1 (uint8)'}  outputporttype=[3]  outputportwidth=[1]  outputportlabel={'Status'}  compat=0  optionstring="[\"1\",\"2\",\"0\",\"0\",\"off\",\"1\"]"
  Terminator : Terminator
  Terminator1 : Terminator
  Terminator2 : Terminator
  VAL : Constant  Value=7  OutDataTypeMode=uint8  OutDataType=fixdt(1, 16)  OutScaling=2^0  OutDataTypeStr=uint8
  VAL1 : Constant  Value=hex2dec('39')  OutDataTypeMode=uint8  OutDataType=fixdt(1, 16)  OutScaling=2^0  OutDataTypeStr=uint8
  VAL2 : Constant  Value=hex2dec('38')  OutDataTypeMode=uint8  OutDataType=fixdt(1, 16)  OutScaling=2^0  OutDataTypeStr=uint8
  wires:
  Soft I2C Master Read/Write2/1 -> Terminator2/1
  VAL1/1 -> Soft I2C Master Read/Write2/3
  PT_DATA_CFG2/1 -> Soft I2C Master Read/Write2/2
  Soft I2C Master Read/Write/1 -> Terminator1/1
  VAL2/1 -> Soft I2C Master Read/Write/3
  PT_DATA_CFG1/1 -> Soft I2C Master Read/Write/2
  Soft I2C Master Read/Write1/1 -> Terminator/1
  VAL/1 -> Soft I2C Master Read/Write1/3
  SlvAddr/1 -> Soft I2C Master Read/Write1/1, Soft I2C Master Read/Write2/1, Soft I2C Master Read/Write/1
  PT_DATA_CFG/1 -> Soft I2C Master Read/Write1/2
